simulink library "AeroLib"  (Simulink 6.0)
settings: Solver=ode45  SolverMode=SingleTasking  StartTime=0.0  StopTime=10.0  RelTol=1e-3
undefined symbols (not defined in the file): Aero, Ap, Atm, Control, Controls, Eng, Flight_cg, Flight_DamperON, Flight_delta_isa, Flight_DeltaSpiral, Flight_InertiaSelect, Flight_ixx, Flight_ixz, Flight_iyy, Flight_izz, Flight_latitude, Flight_LoiterLenght, Flight_LoiterMode, Flight_LoiterRadius, Flight_longitude, Flight_MaxTargetPoints, Flight_SensorsON, Flight_TimeStep, Flight_TowerWind_X, Flight_TowerWind_Y, Flight_TowerWind_Z, Flight_TowerWindON, Flight_Trimming, Flight_TurbON, Flight_weight, Flight_WindGustON, Flight_WindShearON, Flight_ycg, Flight_zcg, Geom, Lgear, Mass, PEG_CDwbnp, PEG_CLht, PEG_CLht_elev, PEG_CLwbnp, PEG_CMht, PEG_CMwbnp, PEG_CNbeta, PEG_CNr, PEG_CNrud, PEG_CRail, PEG_CRbeta, PEG_CRp, PEG_CRrud, PEG_CYbeta, PEG_CYrud, pow, Sensors
libraries: AeroLib x133, simulink3 x49, simulink x37, aerospace x11
(part 3 of 7)

== system AeroLib/Propulsion/Piston_Engine ==
  FeedBack : Inport  Port=1  LatchInput=off
  From_Atmos : Inport  Port=2  LatchInput=off
  Throttle : Inport  Port=3  LatchInput=off
  From_Reset : Inport  Port=4  LatchInput=off
  Fuel_Cut : Inport  Port=5  LatchInput=off
  AVGAS100_Density : Gain  Gain=0.7  SaturateOnIntegerOverflow=on
  Altitude_delta : Fcn  Expr=1.11*sqrt(1/u(1))*u(2) - 0.11
  Bus Selector2 : BusSelector  DialogController=Simulink.DDGSource_Bus  OutputSignals=T_T0,P_P0
  Constant3 : Constant  Value=0
  Constant5 : Constant  Value=0
  Constant6 : Constant  Value=Eng.Fuel.mass
  Fcn : Fcn  Expr=1-u
  Fuel_Flow_Kgps : simulink/Lookup Tables/Interpolation (n-D) using PreLookup  numDimsPopupSelect=1  explicitNumDims=2  table=Eng.Cons  interpMethod=Linear  extrapMethod=Linear  rangeErrorMode=None  NumSelectionDims=0
  Max_Available_Power : simulink/Lookup Tables/Interpolation (n-D) using PreLookup  numDimsPopupSelect=1  explicitNumDims=2  table=Eng.power  interpMethod=Linear  extrapMethod=Linear  rangeErrorMode=None  NumSelectionDims=0
  Mux5 : Mux  Inputs=2
  Product1 : Product  SaturateOnIntegerOverflow=on  InputSameDT=on
  Product2 : Product  SaturateOnIntegerOverflow=on  InputSameDT=on
  Rot_par_min : Fcn  Expr=Eng.MaxRpm*u
  Saturation : Saturate  UpperLimit=Eng.MaxRpm  LowerLimit=Eng.MinRpm
  Stateless_LimIntegrator : AeroLib/AMS_StatelessFilters/Stateless_LimIntegrator
  Sum : Sum  Inputs=++|  SaturateOnIntegerOverflow=on  InputSameDT=on
  Turn : simulink/Lookup Tables/PreLookup Index Search  bpData=Eng.Rpm  searchMode=Binary Search  cacheBpFlag=off  outputFlag=off  IndexDataType=uint32  extrapMode=Linear Extrapolation  rangeErrorMode=None
  Avail_Power : Outport
  RPM : Outport  Port=2
  Fuel_Mass : Outport  Port=3
  wires:
  Fcn/1 -> Product1/2
  Fuel_Flow_Kgps/1 -> Product1/1
  Product1/1 -> AVGAS100_Density/1
  Fuel_Cut/1 -> Fcn/1
  Turn/1 -> Max_Available_Power/1, Fuel_Flow_Kgps/1
  Mux5/1 -> Altitude_delta/1
  Max_Available_Power/1 -> Product2/1
  Altitude_delta/1 -> Product2/2
  Bus Selector2/2 -> Mux5/2  "<P_P0>"
  Bus Selector2/1 -> Mux5/1  "<T_T0>"
  Throttle/1 -> Rot_par_min/1
  Saturation/1 -> Turn/1, RPM/1
  Rot_par_min/1 -> Sum/2
  Sum/1 -> Saturation/1
  FeedBack/1 -> Sum/1
  Product2/1 -> Avail_Power/1
  From_Atmos/1 -> Bus Selector2/1
  AVGAS100_Density/1 -> Stateless_LimIntegrator/3
  Constant3/1 -> Stateless_LimIntegrator/2
  From_Reset/1 -> Stateless_LimIntegrator/1
  Stateless_LimIntegrator/1 -> Fuel_Mass/1
  Constant5/1 -> Stateless_LimIntegrator/4
  Constant6/1 -> Stateless_LimIntegrator/5

== system AeroLib/Propulsion/Piston_Engine_Propeller ==
  From_Atmos : Inport  Port=1  LatchInput=off
  Throttle : Inport  Port=2  LatchInput=off
  From_Reset : Inport  Port=3  LatchInput=off
  Fuel_Cut : Inport  Port=4  LatchInput=off
  Air_Dens : Fcn  Expr=2*u(2)/u(1)^2
  Bus Selector2 : BusSelector  DialogController=Simulink.DDGSource_Bus  OutputSignals=Mach,TAS,DynPres_P
  Fcn : Fcn  Expr=1-u
  Fixed_Pitch_Propeller : AeroLib/Propulsion/Fixed_Pitch_Propeller  reduc=Eng.Prop.reduc  prop_diam=Eng.Prop.diam
  Gain1 : Gain  Gain=Atm.grav  SaturateOnIntegerOverflow=on
  Mux6 : Mux  Inputs=2
  Piston_Engine : AeroLib/Propulsion/Piston_Engine
  Power_Limit : Subsystem
  Product : Product  SaturateOnIntegerOverflow=on  InputSameDT=on
  Propeller_Power_Demand : AeroLib/Propulsion/Propeller_Power_Demand  D=Eng.Prop.diam
  Thrust_N : Outport
  RPM : Outport  Port=2
  Efficiency_coef : Outport  Port=3
  Fuel_Mass : Outport  Port=4
  wires:
  Gain1/1 -> Thrust_N/1
  Fcn/1 -> Product/2
  Product/1 -> Gain1/1
  Fuel_Cut/1 -> Piston_Engine/5, Fcn/1
  From_Reset/1 -> Piston_Engine/4
  Piston_Engine/3 -> Fuel_Mass/1
  Bus Selector2/1 -> Fixed_Pitch_Propeller/2  "<Mach>"
  Bus Selector2/3 -> Mux6/2  "<DynPres_P>"
  Bus Selector2/2 -> Fixed_Pitch_Propeller/3, Mux6/1  "<TAS>"
  Piston_Engine/1 -> Power_Limit/1(Avail_Power)
  Piston_Engine/2 -> Fixed_Pitch_Propeller/1, Power_Limit/2(Rpm), RPM/1
  Throttle/1 -> Piston_Engine/3
  Power_Limit/1(Delta_Rpm) -> Piston_Engine/1
  Propeller_Power_Demand/1 -> Power_Limit/3(Power_Demand)
  Fixed_Pitch_Propeller/3 -> Propeller_Power_Demand/3
  Fixed_Pitch_Propeller/2 -> Propeller_Power_Demand/2
  Fixed_Pitch_Propeller/1 -> Propeller_Power_Demand/1
  Mux6/1 -> Air_Dens/1
  From_Atmos/1 -> Piston_Engine/2, Bus Selector2/1
  Propeller_Power_Demand/2 -> Product/1
  Fixed_Pitch_Propeller/4 -> Efficiency_coef/1
  Air_Dens/1 -> Propeller_Power_Demand/4

== system AeroLib/Propulsion/Piston_Engine_Propeller_system ==
  note: These blocks is included to allow model to be used
      | with DINAMO.
      | DINAMO's Trim capabilities need the model
      | to contain a twin engine type of propulsion system.
  From_Atmos : Inport  Port=1  LatchInput=off
  From_Ctrl : Inport  Port=2  LatchInput=off
  From_Inputs : Inport  Port=3  LatchInput=off
  From_Reset : Inport  Port=4  LatchInput=off
  Booster : AeroLib/Propulsion/Booster  Booster_Time=Eng.Booster.Time  Xpos=Geom.Eng.Booster.Xpos  Ypos=Geom.Eng.Booster.Ypos  Zpos=Geom.Eng.Booster.Zpos  Booster_Thrust=Eng.Booster.Thrust  pitch=Geom.Eng.Booster.pitch
  Bus Creator : BusCreator  DialogController=Simulink.DDGSource_Bus  Inputs=16
  Bus Selector2 : BusSelector  DialogController=Simulink.DDGSource_Bus  OutputSignals=DynPres_P
  Bus Selector3 : BusSelector  DialogController=Simulink.DDGSource_Bus  OutputSignals=FuelCut_LH,FuelCut_RH,BoosterON
  Engine_Transient : AeroLib/Propulsion/Engine_Transient
  Fantom_Engine : Gain  Gain=eps  SaturateOnIntegerOverflow=on
  Fantom_Engine1 : Gain  Gain=eps  SaturateOnIntegerOverflow=on
  Piston_Engine_Propeller_LH : AeroLib/Propulsion/Piston_Engine_Propeller
  Piston_Engine_Propeller_RH : AeroLib/Propulsion/Piston_Engine_Propeller
  Terminator2 : Terminator
  Terminator3 : Terminator
  Thrust_Components : AeroLib/Propulsion/Thrust_Components  grav=Atm.grav  Sw=Geom.Wing.sw  Xpos=Geom.Eng.Xpos  Ypos=Geom.Eng.Ypos  Zpos=Geom.Eng.Zpos  pitch=Geom.Eng.pitch  toeout=Geom.Eng.toeout
  Prop_Out : Outport
  wires:
  Bus Selector2/1 -> Thrust_Components/4  "<DynPres_P>"
  Thrust_Components/12 -> Bus Creator/14  "RH_Throttle"
  Thrust_Components/11 -> Bus Creator/13  "LH_Throttle"
  Piston_Engine_Propeller_LH/4 -> Thrust_Components/2
  From_Atmos/1 -> Piston_Engine_Propeller_RH/1, Piston_Engine_Propeller_LH/1, Bus Selector2/1
  Thrust_Components/9 -> Bus Creator/11  "Thrust_N"
  Thrust_Components/10 -> Bus Creator/12  "DeltaThr"
  Thrust_Components/8 -> Bus Creator/10  "Thrust_Kgf"
  Thrust_Components/7 -> Bus Creator/9  "CT"
  Thrust_Components/6 -> Bus Creator/8  "Nthrust"
  Thrust_Components/5 -> Bus Creator/7  "Mthrust"
  Bus Creator/1 -> Prop_Out/1
  Thrust_Components/1 -> Bus Creator/3  "Xthrust"
  Thrust_Components/4 -> Bus Creator/6  "Lthrust"
  Thrust_Components/3 -> Bus Creator/5  "Zthrust"
  Thrust_Components/2 -> Bus Creator/4  "Ythrust"
  From_Ctrl/1 -> Engine_Transient/1
  From_Inputs/1 -> Bus Selector3/1
  From_Reset/1 -> Piston_Engine_Propeller_LH/3, Piston_Engine_Propeller_RH/3, Booster/2, Engine_Transient/2
  Piston_Engine_Propeller_RH/1 -> Fantom_Engine/1
  Piston_Engine_Propeller_RH/4 -> Fantom_Engine1/1
  Piston_Engine_Propeller_RH/3 -> Terminator2/1
  Booster/1 -> Thrust_Components/8
  Booster/2 -> Bus Creator/16  "StopBooster"
  Engine_Transient/1 -> Piston_Engine_Propeller_LH/2, Thrust_Components/3
  Engine_Transient/2 -> Piston_Engine_Propeller_RH/2, Thrust_Components/7
  Piston_Engine_Propeller_LH/1 -> Thrust_Components/1
  Fantom_Engine/1 -> Thrust_Components/5
  Thrust_Components/13 -> Bus Creator/15  "Fuel_Mass"
  Fantom_Engine1/1 -> Thrust_Components/6
  Piston_Engine_Propeller_LH/2 -> Bus Creator/1  "Rpm_Eng"
  Piston_Engine_Propeller_LH/3 -> Bus Creator/2  "Effic_Prop"
  Bus Selector3/1 -> Piston_Engine_Propeller_LH/4  "<FuelCut_LH>"
  Bus Selector3/2 -> Piston_Engine_Propeller_RH/4  "<FuelCut_RH>"
  Bus Selector3/3 -> Booster/1  "<BoosterON>"
  Piston_Engine_Propeller_RH/2 -> Terminator3/1

== system AeroLib/Propulsion/Propeller_Power_Demand ==
  note: in kg/m3
  note: in hp
  Thrust_coef : Inport  Port=1  LatchInput=off
  Power_coef : Inport  Port=2  LatchInput=off
  Propeller_rps : Inport  Port=3  LatchInput=off
  Air_density : Inport  Port=4  LatchInput=off
  Mux2 : Mux
  N-->Kg : Gain  Gain=1/Atm.grav  SaturateOnIntegerOverflow=on
  Propeller_Power_Demand : Fcn  Expr=u(2)*u(4)*u(3)^3*D^5/75
  Propeller_Trust : Fcn  Expr=u(1)*u(4)*u(3)^2*D^4
  Power_demand : Outport
  Thrust_kgf : Outport  Port=2
  wires:
  Mux2/1 -> Propeller_Trust/1, Propeller_Power_Demand/1
  Thrust_coef/1 -> Mux2/1
  Power_coef/1 -> Mux2/2
  Propeller_rps/1 -> Mux2/3
  Air_density/1 -> N-->Kg/1
  Propeller_Power_Demand/1 -> Power_demand/1
  Propeller_Trust/1 -> Thrust_kgf/1
  N-->Kg/1 -> Mux2/4

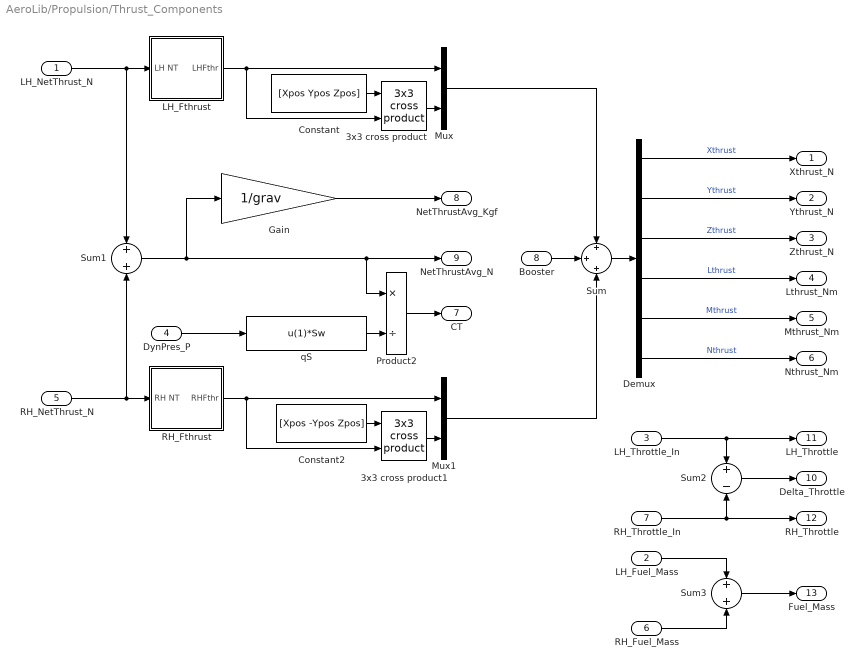
== system AeroLib/Propulsion/Thrust_Components ==
  LH_NetThrust_N : Inport  Port=1  LatchInput=off
  LH_Fuel_Mass : Inport  Port=2  LatchInput=off
  LH_Throttle_In : Inport  Port=3  LatchInput=off
  DynPres_P : Inport  Port=4  LatchInput=off
  RH_NetThrust_N : Inport  Port=5  LatchInput=off
  RH_Fuel_Mass : Inport  Port=6  LatchInput=off
  RH_Throttle_In : Inport  Port=7  LatchInput=off
  Booster : Inport  Port=8  LatchInput=off
  3x3 cross product : aerospace/Axes Transformations/3x3 cross product
  3x3 cross product1 : aerospace/Axes Transformations/3x3 cross product
  Constant : Constant  Value=[Xpos Ypos Zpos]
  Constant2 : Constant  Value=[Xpos -Ypos Zpos]
  Demux : Demux  Outputs=6
  Gain : Gain  Gain=1/grav  SaturateOnIntegerOverflow=on
  LH_Fthrust : Subsystem
  Mux : Mux  Inputs=2
  Mux1 : Mux  Inputs=2
  Product2 : Product  Inputs=*/  SaturateOnIntegerOverflow=on  InputSameDT=on
  RH_Fthrust : Subsystem
  Sum : Sum  Inputs=+|+|+  SaturateOnIntegerOverflow=on  InputSameDT=on
  Sum1 : Sum  SaturateOnIntegerOverflow=on  InputSameDT=on
  Sum2 : Sum  Inputs=+-  SaturateOnIntegerOverflow=on  InputSameDT=on
  Sum3 : Sum  SaturateOnIntegerOverflow=on  InputSameDT=on
  qS : Fcn  Expr=u(1)*Sw
  Xthrust_N : Outport
  Ythrust_N : Outport  Port=2
  Zthrust_N : Outport  Port=3
  Lthrust_Nm : Outport  Port=4
  Mthrust_Nm : Outport  Port=5
  Nthrust_Nm : Outport  Port=6
  CT : Outport  Port=7
  NetThrustAvg_Kgf : Outport  Port=8
  NetThrustAvg_N : Outport  Port=9
  Delta_Throttle : Outport  Port=10
  LH_Throttle : Outport  Port=11
  RH_Throttle : Outport  Port=12
  Fuel_Mass : Outport  Port=13
  wires:
  Sum3/1 -> Fuel_Mass/1
  RH_Fuel_Mass/1 -> Sum3/2
  LH_Fuel_Mass/1 -> Sum3/1
  Gain/1 -> NetThrustAvg_Kgf/1
  DynPres_P/1 -> qS/1
  RH_Throttle_In/1 -> RH_Throttle/1, Sum2/2
  LH_Throttle_In/1 -> LH_Throttle/1, Sum2/1
  Sum1/1 -> Gain/1, Product2/1, NetThrustAvg_N/1
  Booster/1 -> Sum/2
  Constant2/1 -> 3x3 cross product1/1
  3x3 cross product1/1 -> Mux1/2
  Mux1/1 -> Sum/3
  RH_NetThrust_N/1 -> Sum1/2, RH_Fthrust/1(RH NT)
  RH_Fthrust/1(RHFthr) -> 3x3 cross product1/2, Mux1/1
  Sum2/1 -> Delta_Throttle/1
  Demux/1 -> Xthrust_N/1  "Xthrust"
  Demux/6 -> Nthrust_Nm/1  "Nthrust"
  Demux/5 -> Mthrust_Nm/1  "Mthrust"
  Demux/4 -> Lthrust_Nm/1  "Lthrust"
  Demux/3 -> Zthrust_N/1  "Zthrust"
  Demux/2 -> Ythrust_N/1  "Ythrust"
  Constant/1 -> 3x3 cross product/1
  3x3 cross product/1 -> Mux/2
  Mux/1 -> Sum/1
  Product2/1 -> CT/1
  qS/1 -> Product2/2
  LH_NetThrust_N/1 -> Sum1/1, LH_Fthrust/1(LH NT)
  LH_Fthrust/1(LHFthr) -> Mux/1, 3x3 cross product/2
  Sum/1 -> Demux/1

== system AeroLib/Propulsion/Twin_Jet_Engine_system ==
  From_Atmos : Inport  Port=1  LatchInput=off
  From_Ctrl : Inport  Port=2  LatchInput=off
  From_Inputs : Inport  Port=3  LatchInput=off
  From_Reset : Inport  Port=4  LatchInput=off
  Booster : AeroLib/Propulsion/Booster  Booster_Time=Eng.Booster.Time  Xpos=Geom.Eng.Booster.Xpos  Ypos=Geom.Eng.Booster.Ypos  Zpos=Geom.Eng.Booster.Zpos  Booster_Thrust=Eng.Booster.Thrust  pitch=Geom.Eng.Booster.pitch
  Bus Selector1 : BusSelector  DialogController=Simulink.DDGSource_Bus  OutputSignals=DynPres_P
  Bus Selector3 : BusSelector  DialogController=Simulink.DDGSource_Bus  OutputSignals=FuelCut_LH,FuelCut_RH,BoosterON
  Engine_Transient : AeroLib/Propulsion/Engine_Transient
  Jet_Engine_LH : AeroLib/Propulsion/Jet_Engine
  Jet_Engine_RH : AeroLib/Propulsion/Jet_Engine
  Mux : Mux  Inputs=14
  Thrust_Components : AeroLib/Propulsion/Thrust_Components  grav=Atm.grav  Sw=Geom.Wing.sw  Xpos=Geom.Eng.Xpos  Ypos=Geom.Eng.Ypos  Zpos=Geom.Eng.Zpos  pitch=Geom.Eng.pitch  toeout=Geom.Eng.toeout
  Prop_Out : Outport
  wires:
  From_Atmos/1 -> Jet_Engine_LH/2, Jet_Engine_RH/2, Bus Selector1/1
  Engine_Transient/2 -> Jet_Engine_RH/1
  From_Inputs/1 -> Bus Selector3/1
  Booster/2 -> Mux/14  "StopBooster"
  Thrust_Components/2 -> Mux/2  "Ythrust"
  Thrust_Components/3 -> Mux/3  "Zthrust"
  Thrust_Components/4 -> Mux/4  "Lthrust"
  Thrust_Components/1 -> Mux/1  "Xthrust"
  Thrust_Components/5 -> Mux/5  "Mthrust"
  Thrust_Components/6 -> Mux/6  "Nthrust"
  Thrust_Components/7 -> Mux/7  "CT"
  Thrust_Components/8 -> Mux/8  "Thrust_Kgf"
  Thrust_Components/10 -> Mux/10  "DeltaThr"
  Thrust_Components/9 -> Mux/9  "Thrust_N"
  Mux/1 -> Prop_Out/1
  Jet_Engine_RH/3 -> Thrust_Components/7
  Jet_Engine_RH/1 -> Thrust_Components/5
  Booster/1 -> Thrust_Components/8
  Jet_Engine_LH/3 -> Thrust_Components/3
  Jet_Engine_LH/1 -> Thrust_Components/1
  Thrust_Components/13 -> Mux/13  "Fuel_Mass"
  Jet_Engine_LH/2 -> Thrust_Components/2
  Jet_Engine_RH/2 -> Thrust_Components/6
  From_Ctrl/1 -> Engine_Transient/1
  From_Reset/1 -> Jet_Engine_RH/4, Jet_Engine_LH/4, Booster/2, Engine_Transient/2
  Engine_Transient/1 -> Jet_Engine_LH/1
  Thrust_Components/11 -> Mux/11  "RH_Throttle"
  Bus Selector3/1 -> Jet_Engine_LH/3  "<FuelCut_LH>"
  Bus Selector3/2 -> Jet_Engine_RH/3  "<FuelCut_RH>"
  Bus Selector3/3 -> Booster/1  "<BoosterON>"
  Thrust_Components/12 -> Mux/12  "LH_Throttle"
  Bus Selector1/1 -> Thrust_Components/4  "<DynPres_P>"

== system AeroLib/Propulsion/Variable_Pitch_Propeller ==
  note: deg
  RPM : Inport  Port=1  LatchInput=off
  Mach : Inport  Port=2  LatchInput=off
  TAS_mps : Inport  Port=3  LatchInput=off
  PropPitch : Inport  Port=4  LatchInput=off
  Advance_Ratio : Fcn  Expr=u(1)/(prop_diam*u(2))
  Beta : simulink/Lookup Tables/PreLookup Index Search  bpData=Eng.Prop.Beta  searchMode=Binary Search  cacheBpFlag=off  outputFlag=off  IndexDataType=uint32  extrapMode=Linear Extrapolation  rangeErrorMode=None
  CP : simulink/Lookup Tables/Interpolation (n-D) using PreLookup  numDimsPopupSelect=2  explicitNumDims=2  table=Eng.Prop.Cp  interpMethod=Linear  extrapMethod=Linear  rangeErrorMode=None  NumSelectionDims=0
  CT : simulink/Lookup Tables/Interpolation (n-D) using PreLookup  numDimsPopupSelect=2  explicitNumDims=2  table=Eng.Prop.Ct  interpMethod=Linear  extrapMethod=Linear  rangeErrorMode=None  NumSelectionDims=0
  J : simulink/Lookup Tables/PreLookup Index Search  bpData=Eng.Prop.J  searchMode=Binary Search  cacheBpFlag=off  outputFlag=off  IndexDataType=uint32  extrapMode=Linear Extrapolation  rangeErrorMode=None
  Mach_Number_Effect : Subsystem
  Mux1 : Mux  Inputs=2
  Product1 : Product  Inputs=**/  SaturateOnIntegerOverflow=on  InputSameDT=on
  Product2 : Product  Inputs=*/  SaturateOnIntegerOverflow=on  InputSameDT=on
  Product4 : Product  SaturateOnIntegerOverflow=on  InputSameDT=on
  Reduction : Gain  Gain=1/reduc/60  SaturateOnIntegerOverflow=on
  Thrust_coef : Outport
  Power_coef : Outport  Port=2
  Propeller_rps : Outport  Port=3
  Efficiency_coef : Outport  Port=4
  wires:
  PropPitch/1 -> Mach_Number_Effect/5(Prop_Pitch_deg), Beta/1
  Beta/1 -> ?
  J/1 -> CT/1, CP/1
  Mux1/1 -> Advance_Ratio/1
  CP/1 -> Product2/1
  Reduction/1 -> Mux1/2, Propeller_rps/1, Mach_Number_Effect/2(Prop_rps)
  TAS_mps/1 -> Mux1/1, Mach_Number_Effect/3(TAS)
  RPM/1 -> Reduction/1
  Product1/1 -> Efficiency_coef/1
  Mach/1 -> Mach_Number_Effect/4(Mach)
  Product2/1 -> Power_coef/1, Product1/3
  Mach_Number_Effect/2(Kcp) -> Product2/2
  CT/1 -> Product4/1
  Product4/1 -> Product1/1, Thrust_coef/1
  Mach_Number_Effect/1(Km) -> Product4/2
  Advance_Ratio/1 -> Product1/2, J/1, Mach_Number_Effect/1(J)

== system AeroLib/Sensors/Air_Data_Computer ==
  From_Atmos : Inport  Port=1  LatchInput=off
  From_Reset : Inport  Port=2  LatchInput=off
  Bus Selector1 : BusSelector  DialogController=Simulink.DDGSource_Bus  OutputSignals=Pamb_P,DynPres_P,OAT_degC,PresAlt_ft
  Gain2 : Gain  SaturateOnIntegerOverflow=on
  Gain3 : Gain  SaturateOnIntegerOverflow=on
  Gain4 : Gain  SaturateOnIntegerOverflow=on
  Mux : Mux
  Mux1 : Mux  Inputs=3
  SensorsOFF : Subsystem
  Simple_Sensor : AeroLib/Sensors/Simple_Sensor  Var=Sensors.ADC.Var  Seed=Sensors.ADC.Seed  Max=60000  Min=-300  Time_Const=Sensors.ADC.TimeConst
  Sum : Sum  Inputs=++|  SaturateOnIntegerOverflow=on  InputSameDT=on
  Switch : Switch  Threshold=0.5  SaturateOnIntegerOverflow=on  InputSameDT=on
  Ts*Ps/Pt : Fcn  Expr=u(3) * u(2) / u(1)
  ADC_Out : Outport
  wires:
  Simple_Sensor/1 -> Switch/3
  From_Reset/1 -> Simple_Sensor/3
  Switch/1 -> Mux/4  "ADC_PresAlt_ft"
  SensorsOFF/1(SensorsOFF) -> Switch/2
  Bus Selector1/1 -> Sum/1, Gain2/1, Mux1/2  "<Pamb_P>"
  Ts*Ps/Pt/1 -> Gain3/1
  Mux1/1 -> Ts*Ps/Pt/1
  Bus Selector1/3 -> Mux1/3  "<OAT_degC>"
  Bus Selector1/2 -> Sum/2  "<DynPres_P>"
  Sum/1 -> Mux1/1, Gain4/1  "Pt"
  Gain2/1 -> Mux/1  "ADC_Pamb_P"
  Gain3/1 -> Mux/3  "ADC_OAT_degC"
  Gain4/1 -> Mux/2  "ADC_DynlPres_P"
  Mux/1 -> ADC_Out/1
  From_Atmos/1 -> Bus Selector1/1
  Bus Selector1/4 -> Switch/1, Simple_Sensor/1, Simple_Sensor/2  "<PresAlt_ft>"

== system AeroLib/Sensors/Flight_System_Computer ==
  From_IRU : Inport  Port=1  LatchInput=off
  From_GPS : Inport  Port=2  LatchInput=off
  From_ADC : Inport  Port=3  LatchInput=off
  Bus Creator : BusCreator  DialogController=Simulink.DDGSource_Bus  Inputs=26
  Bus Selector1 : BusSelector  DialogController=Simulink.DDGSource_Bus  OutputSignals=IRU_Alpha,IRU_Beta,IRU_KIAS,IRU_TAS_kt,IRU_RadarAlt_ft,IRU_Phi_deg,IRU_Q_degps,IRU_P_degps,IRU_R_degps,IRU_LongAcc_g,IRU_NormAcc_g,IRU_LatAcc_g,IRU_Theta_deg,IRU_HeadMag_deg,IRU_FPath_deg
  Bus Selector4 : BusSelector  DialogController=Simulink.DDGSource_Bus  OutputSignals=IRU_Xdist_m,IRU_Ydist_m,IRU_Latitude_deg,IRU_Longitude_deg,IRU_GeodHeight_m,IRU_VN_kt,IRU_VE_kt,IRU_VD_mps,IRU_GrSpeed_kt,IRU_TrackMag_deg
  Bus Selector5 : BusSelector  DialogController=Simulink.DDGSource_Bus  OutputSignals=GPS_Xdist_m,GPS_Ydist_m,GPS_Latitude_deg,GPS_Longitude_deg,GPS_GeodHeight_m,GPS_VN_kt,GPS_VE_kt,GPS_VD_mps,GPS_Vground_kt,GPS_Track_deg
  Bus Selector6 : BusSelector  DialogController=Simulink.DDGSource_Bus  OutputSignals=ADC_PresAlt_ft
  Bus Selector7 : BusSelector  DialogController=Simulink.DDGSource_Bus  OutputSignals=IRU_PresAlt_ft
  Demux : Demux  Outputs=10
  Gain : Gain  Gain=Kins  SaturateOnIntegerOverflow=on
  Gain1 : Gain  Gain=0.5  SaturateOnIntegerOverflow=on
  Gain2 : Gain  Gain=Kgps  SaturateOnIntegerOverflow=on
  Mux1 : Mux  Inputs=10
  Mux2 : Mux  Inputs=10
  Sum : Sum  Inputs=|++  SaturateOnIntegerOverflow=on  InputSameDT=on
  Sum1 : Sum  Inputs=|++  SaturateOnIntegerOverflow=on  InputSameDT=on
  FSC_Out : Outport
  wires:
  Bus Selector1/15 -> Bus Creator/26  "<IRU_FPath_deg>"
  Bus Selector1/14 -> Bus Creator/25  "<IRU_HeadMag_deg>"
  Bus Selector1/13 -> Bus Creator/24  "<IRU_Theta_deg>"
  Bus Creator/1 -> FSC_Out/1
  Bus Selector1/12 -> Bus Creator/23  "<IRU_LatAcc_g>"
  Bus Selector1/11 -> Bus Creator/22  "<IRU_NormAcc_g>"
  Bus Selector1/10 -> Bus Creator/21  "<IRU_LongAcc_g>"
  Bus Selector1/9 -> Bus Creator/20  "<IRU_R_degps>"
  Bus Selector1/8 -> Bus Creator/19  "<IRU_P_degps>"
  Bus Selector1/7 -> Bus Creator/18  "<IRU_Q_degps>"
  Bus Selector1/6 -> Bus Creator/17  "<IRU_Phi_deg>"
  Bus Selector1/5 -> Bus Creator/16  "<IRU_RadarAlt_ft>"
  Bus Selector1/4 -> Bus Creator/15  "<IRU_TAS_kt>"
  Bus Selector1/3 -> Bus Creator/14  "<IRU_KIAS>"
  Bus Selector1/2 -> Bus Creator/13  "<IRU_Beta>"
  Bus Selector1/1 -> Bus Creator/12  "<IRU_Alpha>"
  Gain1/1 -> Bus Creator/1  "FSC_Altitude_ft"
  Demux/10 -> Bus Creator/11  "FSC_TrackMag_deg"
  Demux/9 -> Bus Creator/10  "FSC_GrSpeed_kt"
  Demux/8 -> Bus Creator/9  "FSC_VD_mps"
  Demux/7 -> Bus Creator/8  "FSC_VE_kt"
  Demux/6 -> Bus Creator/7  "FSC_VN_kt"
  Demux/5 -> Bus Creator/6  "FSC_GeodHeight_m"
  Demux/4 -> Bus Creator/5  "FSC_Longitude_deg"
  Demux/3 -> Bus Creator/4  "FSC_Latitude_deg"
  Demux/2 -> Bus Creator/3  "FSC_Ydist_m"
  Demux/1 -> Bus Creator/2  "FSC_Xdist_m"
  Sum/1 -> Demux/1
  Sum1/1 -> Gain1/1
  Bus Selector7/1 -> Sum1/2  "<IRU_PresAlt_ft>"
  Bus Selector6/1 -> Sum1/1  "<ADC_PresAlt_ft>"
  Bus Selector4/10 -> Mux2/10  "<IRU_TrackMag_deg>"
  Bus Selector4/9 -> Mux2/9  "<IRU_GrSpeed_kt>"
  Bus Selector4/8 -> Mux2/8  "<IRU_VD_mps>"
  Bus Selector4/7 -> Mux2/7  "<IRU_VE_kt>"
  Bus Selector4/6 -> Mux2/6  "<IRU_VN_kt>"
  Bus Selector4/5 -> Mux2/5  "<IRU_GeodHeight_m>"
  Bus Selector4/4 -> Mux2/4  "<IRU_Longitude_deg>"
  Bus Selector4/3 -> Mux2/3  "<IRU_Latitude_deg>"
  Bus Selector4/2 -> Mux2/2  "<IRU_Ydist_m>"
  Bus Selector4/1 -> Mux2/1  "<IRU_Xdist_m>"
  Bus Selector5/10 -> Mux1/10  "<GPS_Track_deg>"
  Bus Selector5/9 -> Mux1/9  "<GPS_Vground_kt>"
  Bus Selector5/8 -> Mux1/8  "<GPS_VD_mps>"
  Bus Selector5/7 -> Mux1/7  "<GPS_VE_kt>"
  Bus Selector5/6 -> Mux1/6  "<GPS_VN_kt>"
  Bus Selector5/5 -> Mux1/5  "<GPS_GeodHeight_m>"
  Bus Selector5/4 -> Mux1/4  "<GPS_Longitude_deg>"
  Bus Selector5/3 -> Mux1/3  "<GPS_Latitude_deg>"
  Bus Selector5/2 -> Mux1/2  "<GPS_Ydist_m>"
  Bus Selector5/1 -> Mux1/1  "<GPS_Xdist_m>"
  Gain2/1 -> Sum/2
  Gain/1 -> Sum/1
  Mux1/1 -> Gain2/1
  Mux2/1 -> Gain/1
  From_IRU/1 -> Bus Selector1/1, Bus Selector7/1, Bus Selector4/1
  From_ADC/1 -> Bus Selector6/1
  From_GPS/1 -> Bus Selector5/1

== system AeroLib/Sensors/Gauss_Markov ==
  Reset : Inport  Port=1  LatchInput=off
  Constant : Constant  Value=0
  Gain : Gain  Orientation=left  Gain=1/tau  SaturateOnIntegerOverflow=on
  Stateless_Integrator : AeroLib/AMS_StatelessFilters/Stateless_Integrator
  Sum : Sum  Inputs=|+-  SaturateOnIntegerOverflow=on  InputSameDT=on
  White Noise : RandomNumber  Variance=Var  Seed=Seed  SampleTime=Flight_TimeStep
  Noise : Outport
  wires:
  Reset/1 -> Stateless_Integrator/1
  Constant/1 -> Stateless_Integrator/2
  White Noise/1 -> Sum/1
  Sum/1 -> Stateless_Integrator/3
  Stateless_Integrator/1 -> Noise/1, Gain/1
  Gain/1 -> Sum/2

== system AeroLib/Sensors/Global_Positioning_System ==
  Latitude : Inport  Port=1  LatchInput=off
  Longitude : Inport  Port=2  LatchInput=off
  GeodHeight : Inport  Port=3  LatchInput=off
  VN_kt : Inport  Port=4  LatchInput=off
  VE_kt : Inport  Port=5  LatchInput=off
  VD_mps : Inport  Port=6  LatchInput=off
  Xdist_m : Inport  Port=7  LatchInput=off
  Ydist_m : Inport  Port=8  LatchInput=off
  Track_deg : Inport  Port=9  LatchInput=off
  From_Reset : Inport  Port=10  LatchInput=off
  Bus Creator : BusCreator  DialogController=Simulink.DDGSource_Bus  Inputs=10
  Clock : Clock
      settings: Decimation=10
  Constant : Constant  Value=Flight_Trimming
  Demux : Demux  Outputs=9
  Fcn : Fcn  Expr=u <= max(Time_delay)
  Fcn1 : Fcn  Expr=sqrt(u(4)^2 + u(5)^2)
  Mux : Mux  Inputs=9
  SensorsOFF : Subsystem
  Simple_GPS : Subsystem
  Switch : Switch  Threshold=0.5  SaturateOnIntegerOverflow=on  InputSameDT=on
  Switch1 : Switch  Threshold=0.5  SaturateOnIntegerOverflow=on  InputSameDT=on
  or : Logic  Operator=OR
  GPS_Out : Outport
  wires:
  From_Reset/1 -> Simple_GPS/2("From_Reset ")
  Switch1/1 -> Fcn1/1, Demux/1
  Switch/1 -> Switch1/3
  SensorsOFF/1(SensorsOFF) -> Switch1/2
  Clock/1 -> Fcn/1
  Constant/1 -> or/1  "DT"
  Fcn/1 -> or/2
  or/1 -> Switch/2
  Latitude/1 -> Mux/1
  Longitude/1 -> Mux/2
  GeodHeight/1 -> Mux/3
  VN_kt/1 -> Mux/4
  VE_kt/1 -> Mux/5
  VD_mps/1 -> Mux/6
  Simple_GPS/1(GPS_Out) -> Switch/3
  Demux/6 -> Bus Creator/6  "GPS_VD_mps"
  Demux/5 -> Bus Creator/5  "GPS_VE_kt"
  Demux/4 -> Bus Creator/4  "GPS_VN_kt"
  Demux/3 -> Bus Creator/3  "GPS_GeodHeight_m"
  Demux/2 -> Bus Creator/2  "GPS_Longitude_deg"
  Demux/1 -> Bus Creator/1  "GPS_Latitude_deg"
  Mux/1 -> Simple_GPS/1(Measured_In), Switch1/1, Switch/1
  Bus Creator/1 -> GPS_Out/1
  Fcn1/1 -> Bus Creator/10  "GPS_Vground_kt"
  Xdist_m/1 -> Mux/7
  Ydist_m/1 -> Mux/8
  Demux/7 -> Bus Creator/7  "GPS_Xdist_m"
  Demux/8 -> Bus Creator/8  "GPS_Ydist_m"
  Track_deg/1 -> Mux/9
  Demux/9 -> Bus Creator/9  "GPS_Track_deg"

== system AeroLib/Sensors/Inertial_Reference_Unit ==
  From_EQM : Inport  Port=1  LatchInput=off
  From_Atmos : Inport  Port=2  LatchInput=off
  From_Reset : Inport  Port=3  LatchInput=off
  Accelerometers : Subsystem
  Airspeed_Detectors : Subsystem
  Altitude_Sensors : Subsystem
  Flow_Incidence_Angle_Sensors : Subsystem
  Gyrospopes : Subsystem
  Mux : Mux  Inputs=37
  IRU_Out : Outport
  wires:
  From_Reset/1 -> Accelerometers/2(From_Reset), Flow_Incidence_Angle_Sensors/2(From_Reset), Altitude_Sensors/3(From_Reset), Airspeed_Detectors/3(From_Reset)
  From_Atmos/1 -> Altitude_Sensors/1(From_Atmos), Airspeed_Detectors/2(From_Atmos), Flow_Incidence_Angle_Sensors/1(From_Atmos)
  Altitude_Sensors/2(IRU_RadarAlt_ft) -> Mux/37  "IRU_RadarAlt_ft"
  Altitude_Sensors/1(IRU_PresAlt_ft) -> Mux/36  "IRU_PresAlt_ft"
  Flow_Incidence_Angle_Sensors/2(IRU_Beta) -> Mux/35  "IRU_Beta"
  Flow_Incidence_Angle_Sensors/1(IRU_Alpha) -> Mux/34  "IRU_Alpha"
  Airspeed_Detectors/3(IRU_TAS_kt) -> Mux/33  "IRU_TAS_kt"
  Airspeed_Detectors/2(IRU_KIAS) -> Mux/32  "IRU_KIAS"
  Airspeed_Detectors/1(IRU_GrSpeed_kt) -> Mux/31  "IRU_GrSpeed_kt"
  Accelerometers/18(IRU_GeodHeight_m) -> Mux/30  "IRU_GeodHeight_m"
  Accelerometers/17(IRU_Longitude_deg) -> Mux/29  "IRU_Longitude_deg"
  Accelerometers/16(IRU_Latitude_deg) -> Mux/28  "IRU_Latitude_deg"
  Accelerometers/14(IRU_Xdist) -> Mux/26  "IRU_Xdist_m"
  Accelerometers/15(IRU_Ydist) -> Mux/27  "IRU_Ydist_m"
  Accelerometers/13(IRU_VD_mps) -> Mux/25  "IRU_VD_mps"
  Accelerometers/11(IRU_VN_kt) -> Mux/23  "IRU_VN_kt"
  Accelerometers/12(IRU_VE_kt) -> Mux/24  "IRU_VE_kt"
  Accelerometers/9(IRU_AlongHeadAcc_g) -> Mux/21  "IRU_AlongHeadAcc_g"
  Accelerometers/10(IRU_CrossHeadAcc_g) -> Mux/22  "IRU_CrossHeadAcc_g"
  Accelerometers/8(IRU_AbNormAcc_g) -> Mux/20  "IRU_AbNormAcc_g"
  Accelerometers/7(IRU_AlongPathAcc_g) -> Mux/19  "IRU_AlongtPath_g"
  Accelerometers/6(IRU_VertAcc_g) -> Mux/18  "IRU_VertAcc_g"
  Accelerometers/4(IRU_AlongTrackAcc_g) -> Mux/16  "IRU_AlongTrackAcc_g"
  Accelerometers/5(IRU_CrossTrackAcc_g) -> Mux/17  "IRU_CrossTrackAcc_g"
  Accelerometers/1(IRU_LongAcc_g) -> Mux/13  "IRU_LongAcc_g"
  Accelerometers/2(IRU_LatAcc_g) -> Mux/14  "IRU_LatAcc_g"
  Accelerometers/3(IRU_NormAcc_g) -> Mux/15  "IRU_NormAcc_g"
  Gyrospopes/5(IRU_R_degps) -> Mux/5  "IRU_R_degps"
  Gyrospopes/4(IRU_P_degps) -> Mux/4  "IRU_P_degps"
  Gyrospopes/3(IRU_Q_degps) -> Mux/3  "IRU_Q_degps"
  Gyrospopes/2(IRU_Phi_deg) -> Mux/2  "IRU_Phi_deg"
  Gyrospopes/1(IRU_Theta_deg) -> Mux/1  "IRU_Theta_deg"
  From_EQM/1 -> Accelerometers/1(From_EQM), Airspeed_Detectors/1(From_EQM), Altitude_Sensors/2(From_EQM), Gyrospopes/1(From_EQM)
  Gyrospopes/6(IRU_Track_deg) -> Mux/6  "IRU_Track_deg"
  Gyrospopes/7(IRU_Head_deg) -> Mux/7  "IRU_Head_deg"
  Gyrospopes/12(IRU_FPath_deg) -> Mux/12  "IRU_FPath_deg"
  Mux/1 -> IRU_Out/1
  Gyrospopes/8(IRU_TrackMag_deg) -> Mux/8  "IRU_TrackMag_deg"
  Gyrospopes/9(IRU_HeadMag_deg) -> Mux/9  "IRU_HeadMag_deg"
  Gyrospopes/10(IRU_DriftAngle_deg) -> Mux/10  "IRU_DriftAngle_deg"
  Gyrospopes/11(IRU_PlatformHead_deg) -> Mux/11  "IRU_PlatformHead_deg"

== system AeroLib/Sensors/Navigation_Sensors ==
  From_EQM : Inport  Port=1  LatchInput=off
  From_Atmos : Inport  Port=2  LatchInput=off
  From_Reset : Inport  Port=3  LatchInput=off
  Air_Data_Computer : AeroLib/Sensors/Air_Data_Computer
  Bus Selector : BusSelector  DialogController=Simulink.DDGSource_Bus  OutputSignals=Latitude,Longitude,GeodHeight,VN_kt,VE_kt,VD_mps,Xdist_m,Ydist_m,Track_deg
  Flight_System_Computer : AeroLib/Sensors/Flight_System_Computer  Kgps=Sensors.FSC.Kgps  Kins=Sensors.FSC.Kins
  Global_Positioning_System : AeroLib/Sensors/Global_Positioning_System  Time_delay=Sensors.GPS.TimeDelay  Var=Sensors.GPS.Var  Seed=Sensors.GPS.Seed  Time=Sensors.GPS.CorTime
  Inertial_Reference_Unit : AeroLib/Sensors/Inertial_Reference_Unit  PlatformDev=Sensors.IRU.PlatDev  MagDev=Sensors.IRU.MagDev
  IRU_Out : Outport
  GPS_Out : Outport  Port=2
  FSC_Out : Outport  Port=3
  wires:
  Air_Data_Computer/1 -> Flight_System_Computer/3
  Global_Positioning_System/1 -> Flight_System_Computer/2, GPS_Out/1
  Flight_System_Computer/1 -> FSC_Out/1
  Bus Selector/7 -> Global_Positioning_System/7  "<Xdist_m>"
  Bus Selector/8 -> Global_Positioning_System/8  "<Ydist_m>"
  From_Reset/1 -> Global_Positioning_System/10, Inertial_Reference_Unit/3, Air_Data_Computer/2
  Bus Selector/3 -> Global_Positioning_System/3  "<GeodHeight>"
  Bus Selector/4 -> Global_Positioning_System/4  "<VN_kt>"
  Bus Selector/5 -> Global_Positioning_System/5  "<VE_kt>"
  Bus Selector/6 -> Global_Positioning_System/6  "<VD_mps>"
  Bus Selector/2 -> Global_Positioning_System/2  "<Longitude>"
  Bus Selector/1 -> Global_Positioning_System/1  "<Latitude>"
  From_EQM/1 -> Bus Selector/1, Inertial_Reference_Unit/1
  Inertial_Reference_Unit/1 -> Flight_System_Computer/1, IRU_Out/1
  From_Atmos/1 -> Air_Data_Computer/1, Inertial_Reference_Unit/2
  Bus Selector/9 -> Global_Positioning_System/9  "<Track_deg>"

== system AeroLib/Sensors/Random Walk ==
  Reset : Inport  Port=1  LatchInput=off
  Constant : Constant  Value=0
  Stateless_Integrator : AeroLib/AMS_StatelessFilters/Stateless_Integrator
  White Noise : RandomNumber  Variance=Var  Seed=Seed  SampleTime=Flight_TimeStep
  Noise : Outport
  wires:
  Reset/1 -> Stateless_Integrator/1
  Constant/1 -> Stateless_Integrator/2
  White Noise/1 -> Stateless_Integrator/3
  Stateless_Integrator/1 -> Noise/1

== system AeroLib/Sensors/Simple_Sensor ==
  Meas_In : Inport  Port=1  LatchInput=off
  X0 : Inport  Port=2  LatchInput=off
  Reset : Inport  Port=3  LatchInput=off
  Gain1 : Gain  Gain=Time_Const  SaturateOnIntegerOverflow=on
  Random Walk : AeroLib/Sensors/Random Walk  Seed=Seed  Var=Var
  Saturation : Saturate  UpperLimit=Max  LowerLimit=Min
  Stateless_Integrator : AeroLib/AMS_StatelessFilters/Stateless_Integrator
  Sum : Sum  Inputs=|+-  SaturateOnIntegerOverflow=on  InputSameDT=on
  Sum1 : Sum  Inputs=++|  SaturateOnIntegerOverflow=on  InputSameDT=on
  Sen_Out : Outport
  wires:
  Reset/1 -> Stateless_Integrator/1, Random Walk/1
  Random Walk/1 -> Sum1/1
  X0/1 -> Stateless_Integrator/2
  Saturation/1 -> Sum/1
  Stateless_Integrator/1 -> Sum1/2, Sum/2
  Sum/1 -> Gain1/1
  Meas_In/1 -> Saturation/1
  Gain1/1 -> Stateless_Integrator/3
  Sum1/1 -> Sen_Out/1

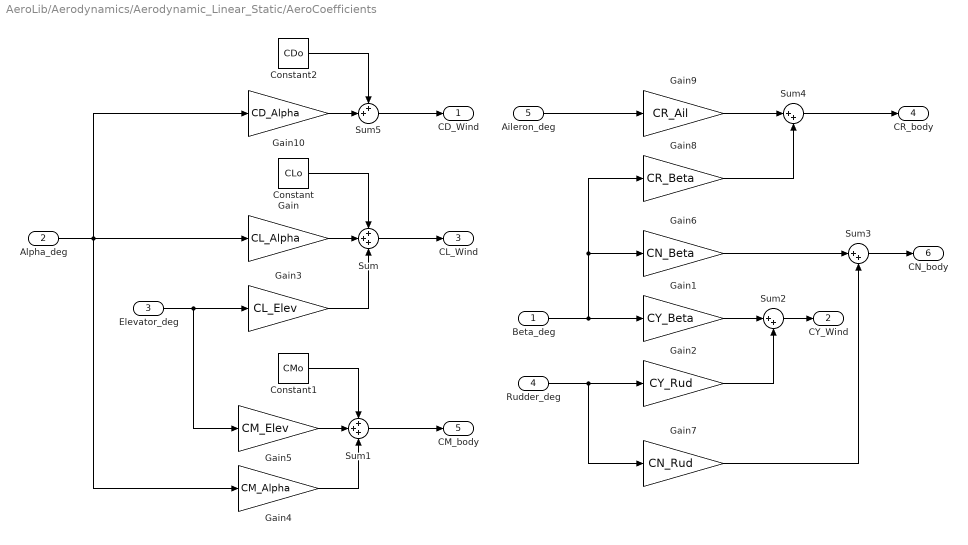
== system AeroLib/Aerodynamics/Aerodynamic_Linear_Static/AeroCoefficients ==
  Beta_deg : Inport  Port=1  LatchInput=off
  Alpha_deg : Inport  Port=2  LatchInput=off
  Elevator_deg : Inport  Port=3  LatchInput=off
  Rudder_deg : Inport  Port=4  LatchInput=off
  Aileron_deg : Inport  Port=5  LatchInput=off
  Constant : Constant  Value=CLo
  Constant1 : Constant  Value=CMo
  Constant2 : Constant  Value=CDo
  Gain : Gain  Gain=CL_Alpha  SaturateOnIntegerOverflow=on
  Gain1 : Gain  Gain=CY_Beta  SaturateOnIntegerOverflow=on
  Gain10 : Gain  Gain=CD_Alpha  SaturateOnIntegerOverflow=on
  Gain2 : Gain  Gain=CY_Rud  SaturateOnIntegerOverflow=on
  Gain3 : Gain  Gain=CL_Elev  SaturateOnIntegerOverflow=on
  Gain4 : Gain  Gain=CM_Alpha  SaturateOnIntegerOverflow=on
  Gain5 : Gain  Gain=CM_Elev  SaturateOnIntegerOverflow=on
  Gain6 : Gain  Gain=CN_Beta  SaturateOnIntegerOverflow=on
  Gain7 : Gain  Gain=CN_Rud  SaturateOnIntegerOverflow=on
  Gain8 : Gain  Gain=CR_Beta  SaturateOnIntegerOverflow=on
  Gain9 : Gain  Gain=CR_Ail  SaturateOnIntegerOverflow=on
  Sum : Sum  Inputs=+++  SaturateOnIntegerOverflow=on
  Sum1 : Sum  Inputs=+++  SaturateOnIntegerOverflow=on
  Sum2 : Sum  Inputs=|++  SaturateOnIntegerOverflow=on
  Sum3 : Sum  Inputs=|++  SaturateOnIntegerOverflow=on
  Sum4 : Sum  Inputs=|++  SaturateOnIntegerOverflow=on
  Sum5 : Sum  Inputs=++|  SaturateOnIntegerOverflow=on
  CD_Wind : Outport
  CY_Wind : Outport  Port=2
  CL_Wind : Outport  Port=3
  CR_body : Outport  Port=4
  CM_body : Outport  Port=5
  CN_body : Outport  Port=6
  wires:
  Constant2/1 -> Sum5/1
  Gain10/1 -> Sum5/2
  Sum5/1 -> CD_Wind/1
  Sum2/1 -> CY_Wind/1
  Sum4/1 -> CR_body/1
  Sum3/1 -> CN_body/1
  Gain9/1 -> Sum4/1
  Gain8/1 -> Sum4/2
  Aileron_deg/1 -> Gain9/1
  Gain7/1 -> Sum3/2
  Gain6/1 -> Sum3/1
  Gain2/1 -> Sum2/2
  Rudder_deg/1 -> Gain7/1, Gain2/1
  Gain1/1 -> Sum2/1
  Beta_deg/1 -> Gain6/1, Gain8/1, Gain1/1
  Constant1/1 -> Sum1/1
  Constant/1 -> Sum/1
  Gain3/1 -> Sum/3
  Gain/1 -> Sum/2
  Sum1/1 -> CM_body/1
  Gain4/1 -> Sum1/3
  Gain5/1 -> Sum1/2
  Elevator_deg/1 -> Gain5/1, Gain3/1
  Sum/1 -> CL_Wind/1
  Alpha_deg/1 -> Gain10/1, Gain/1, Gain4/1

== system AeroLib/Aerodynamics/Aerodynamics_Generic/Aero_Loads ==
  From_Drag : Inport  Port=1  LatchInput=off
  From_SideF : Inport  Port=2  LatchInput=off
  From_Lift : Inport  Port=3  LatchInput=off
  From_Roll : Inport  Port=4  LatchInput=off
  From_Pitch : Inport  Port=5  LatchInput=off
  From_Yaw : Inport  Port=6  LatchInput=off
  From_Atmos : Inport  Port=7  LatchInput=off
  dcg2ac : Inport  Port=8  LatchInput=off
  Bus Selector : BusSelector  DialogController=Simulink.DDGSource_Bus  OutputSignals=DynPres_P,Alpha
  Bus Selector1 : BusSelector  DialogController=Simulink.DDGSource_Bus  OutputSignals=CYs
  Bus Selector2 : BusSelector  DialogController=Simulink.DDGSource_Bus  OutputSignals=CLs
  Demux : Demux  Outputs=6
  Loads : AeroLib/Aerodynamics/Loads  Bref=Geom.Wing.bref  Cref=Geom.Wing.cref  Sw=Geom.Wing.sw
  Mux : Mux  Inputs=10
  Mux1 : Mux  Inputs=6
  STA2BOA : AeroLib/CoordinateSystems/STA2BOA
  Transf to CG : AeroLib/Aerodynamics/Transf to CG  Bref=Geom.Wing.bref  Cref=Geom.Wing.cref
  Xaero : Outport
  wires:
  dcg2ac/1 -> Transf to CG/7
  Demux/6 -> Transf to CG/6
  Demux/5 -> Transf to CG/5
  Demux/4 -> Transf to CG/4
  Demux/3 -> Transf to CG/3
  Demux/2 -> Transf to CG/2
  Demux/1 -> Transf to CG/1
  Transf to CG/6 -> Mux/9, Loads/7  "CNcg"
  Transf to CG/5 -> Mux/8, Loads/6  "CMcg"
  Transf to CG/4 -> Mux/7, Loads/5  "CRcg"
  Transf to CG/3 -> Loads/4
  Transf to CG/2 -> Loads/3
  Transf to CG/1 -> Loads/2
  Bus Selector2/1 -> Mux1/3  "<CLs>"
  Bus Selector1/1 -> Mux1/2  "<CYs>"
  From_Drag/1 -> Mux1/1  "CDs"
  Bus Selector/2 -> STA2BOA/2  "<Alpha>"
  From_Atmos/1 -> Bus Selector/1
  STA2BOA/1 -> Demux/1
  Mux1/1 -> STA2BOA/1, Mux/10  "Caero"
  From_Yaw/1 -> Mux1/6  "CNs"
  From_Pitch/1 -> Mux1/5  "CMs"
  From_Roll/1 -> Mux1/4  "CRs"
  From_Lift/1 -> Bus Selector2/1  "CLs"
  From_SideF/1 -> Bus Selector1/1
  Bus Selector/1 -> Loads/1  "<DynPres_P>"
  Loads/1 -> Mux/1  "Xaero"
  Loads/2 -> Mux/2  "Yaero"
  Loads/3 -> Mux/3  "Zaero"
  Loads/4 -> Mux/4  "Laero"
  Loads/5 -> Mux/5  "Maero"
  Loads/6 -> Mux/6  "Naero"
  Mux/1 -> Xaero/1

== system AeroLib/Aerodynamics/Aerodynamics_Generic/Drag ==
  From_Atmos : Inport  Port=1  LatchInput=off
  From_Ctrl : Inport  Port=2  LatchInput=off
  From_Inputs : Inport  Port=3  LatchInput=off
  " (14)" : Product  Inputs=**  SaturateOnIntegerOverflow=on  InputSameDT=on
  " (15)" : Sum  SaturateOnIntegerOverflow=on  InputSameDT=on
  " (15)1" : Sum  SaturateOnIntegerOverflow=on  InputSameDT=on
  " (22)" : Abs  SaturateOnIntegerOverflow=on
  Bus Selector1 : BusSelector  DialogController=Simulink.DDGSource_Bus  OutputSignals=Alpha,Mach,Beta
  Bus Selector2 : BusSelector  DialogController=Simulink.DDGSource_Bus  OutputSignals=Flap_deg
  Bus Selector3 : BusSelector  DialogController=Simulink.DDGSource_Bus  OutputSignals=GearDown
  CD_wbnp : simulink3/Functions & Tables/Interpolation (n-D) using PreLook-Up  numDimsPopupSelect=3  explicitNumDims=2  table=Aero.Drag.CDs  interpMethod=Linear  extrapMethod=Linear  rangeErrorMode=None
  CdLgAlph : simulink3/Functions & Tables/Look-Up Table (2-D)  x="[-15.0 -10.0  -5.0   0.0   5.0  10.0  15.0  20.0]"  y=[0 10 20 35]  t=Aero.Drag.CDlg
  CdLgBeta : Lookup  DialogController=Simulink.DDGSource  InputValues=[0 5 10 15 20 25 30]  OutputValues="[0.0  0.0008  0.0050  0.0110  0.0190  0.0280 0.0300]"  SaturateOnIntegerOverflow=on
  Gain : Gain  Gain=PEG_CDwbnp  SaturateOnIntegerOverflow=on
  PreLook-Up Index Search3 : simulink3/Functions & Tables/PreLook-Up Index Search  bpData=Aero.Drag.Flap  searchMode=Binary Search  cacheBpFlag=off  outputFlag=off  extrapMode=Linear Extrapolation  rangeErrorMode=None
  PreLook-Up Index Search4 : simulink3/Functions & Tables/PreLook-Up Index Search  bpData=Aero.Drag.Mach  searchMode=Binary Search  cacheBpFlag=off  outputFlag=off  extrapMode=Linear Extrapolation  rangeErrorMode=None
  PreLook-Up Index Search5 : simulink3/Functions & Tables/PreLook-Up Index Search  bpData=Aero.Drag.Alpha  searchMode=Binary Search  cacheBpFlag=off  outputFlag=off  extrapMode=Linear Extrapolation  rangeErrorMode=None
  Drag_Out : Outport
  wires:
  Bus Selector3/1 -> " (14)"/2  "<GearDown>"
  " (15)1"/1 -> Drag_Out/1  "CDs"
  CdLgBeta/1 -> " (15)"/2  "CdLgBeta"
  Bus Selector1/3 -> " (22)"/1  "<Beta>"
  " (22)"/1 -> CdLgBeta/1
  From_Inputs/1 -> Bus Selector3/1
  CdLgAlph/1 -> " (15)"/1  "CDlgAlpha"
  " (15)"/1 -> " (14)"/1
  " (14)"/1 -> " (15)1"/2  "CDlg_A"
  PreLook-Up Index Search5/1 -> CD_wbnp/1
  Bus Selector1/2 -> PreLook-Up Index Search4/1  "<Mach>"
  Bus Selector1/1 -> CdLgAlph/1, PreLook-Up Index Search5/1  "<Alpha>"
  Bus Selector2/1 -> CdLgAlph/2, PreLook-Up Index Search3/1  "<Flap_deg>"
  From_Ctrl/1 -> Bus Selector2/1
  From_Atmos/1 -> Bus Selector1/1
  PreLook-Up Index Search4/1 -> CD_wbnp/3
  PreLook-Up Index Search3/1 -> CD_wbnp/2
  CD_wbnp/1 -> Gain/1  "CDs"
  Gain/1 -> " (15)1"/1

== system AeroLib/Aerodynamics/Aerodynamics_Generic/LIft ==
  From_EQM : Inport  Port=1  LatchInput=off
  From_Atmos : Inport  Port=2  LatchInput=off
  From_Ctrl : Inport  Port=3  LatchInput=off
  Bus Selector : BusSelector  DialogController=Simulink.DDGSource_Bus  OutputSignals=Flap_deg
  Bus Selector1 : BusSelector  DialogController=Simulink.DDGSource_Bus  OutputSignals=Alpha,Mach
  CL Tail : Subsystem
  CL_wnbn : simulink3/Functions & Tables/Interpolation (n-D) using PreLook-Up  numDimsPopupSelect=3  explicitNumDims=2  table=Aero.Lift.CLs  interpMethod=Linear  extrapMethod=Linear  rangeErrorMode=None
  Fcn1 : Fcn  Expr=0.6 + 0.14*u(1) + (0.35 - 0.0045*u(1))*u(2)
  Gain1 : Gain  Gain=PEG_CLwbnp  SaturateOnIntegerOverflow=on
  Mux : Mux  Inputs=2
  Mux1 : Mux  Inputs=2
  PreLook-Up Index Search : simulink3/Functions & Tables/PreLook-Up Index Search  bpData=Aero.Lift.Flap  searchMode=Binary Search  cacheBpFlag=off  outputFlag=off  extrapMode=Linear Extrapolation  rangeErrorMode=None
  PreLook-Up Index Search1 : simulink3/Functions & Tables/PreLook-Up Index Search  bpData=Aero.Lift.Mach  searchMode=Binary Search  cacheBpFlag=off  outputFlag=off  extrapMode=Linear Extrapolation  rangeErrorMode=None
  PreLook-Up Index Search2 : simulink3/Functions & Tables/PreLook-Up Index Search  bpData=Aero.Lift.Alpha  searchMode=Binary Search  cacheBpFlag=off  outputFlag=off  extrapMode=Linear Extrapolation  rangeErrorMode=None
  Sum : Sum  Inputs=+|+  SaturateOnIntegerOverflow=on  InputSameDT=on
  Lift_Out : Outport
  wires:
  From_EQM/1 -> CL Tail/4(From_EQM)
  PreLook-Up Index Search/1 -> CL_wnbn/2
  PreLook-Up Index Search2/1 -> CL_wnbn/1
  Sum/1 -> Mux1/2  "CLs"
  Mux1/1 -> Lift_Out/1  "Lift_s"
  CL Tail/1(CL_Tail) -> Mux1/1, Sum/1  "CLt"
  CL_wnbn/1 -> Gain1/1  "CLwn"
  Fcn1/1 -> CL Tail/2(Epsilon)  "Epsilon"
  Mux/1 -> Fcn1/1
  Bus Selector/1 -> Mux/1, PreLook-Up Index Search/1  "<Flap_deg>"
  Bus Selector1/2 -> PreLook-Up Index Search1/1  "<Mach>"
  Bus Selector1/1 -> Mux/2, PreLook-Up Index Search2/1  "<Alpha>"
  From_Atmos/1 -> CL Tail/3(From_Atmos), Bus Selector1/1
  From_Ctrl/1 -> CL Tail/1(From_Inputs), Bus Selector/1
  PreLook-Up Index Search1/1 -> CL_wnbn/3
  Gain1/1 -> Sum/2  "CLwn"

== system AeroLib/Aerodynamics/Aerodynamics_Generic/Pitching Moment ==
  From_Lift : Inport  Port=1  LatchInput=off
  From_Atmos : Inport  Port=2  LatchInput=off
  From_Ctrl : Inport  Port=3  LatchInput=off
  From_Inputs : Inport  Port=4  LatchInput=off
  " (7)" : Product  Inputs=**  SaturateOnIntegerOverflow=on  InputSameDT=on
  Alpha-Flap Interp1 : simulink3/Functions & Tables/Interpolation (n-D) using PreLook-Up  numDimsPopupSelect=2  explicitNumDims=2  table=Aero.Pitch.CmLG  interpMethod=Linear  extrapMethod=Linear  rangeErrorMode=None
  AlphaIndex : simulink3/Functions & Tables/PreLook-Up Index Search  bpData=[-15 -10 15 20]  searchMode=Linear Search  cacheBpFlag=on  outputFlag=off  extrapMode=Linear Extrapolation  rangeErrorMode=None
  Bus Selector : BusSelector  DialogController=Simulink.DDGSource_Bus  OutputSignals=CLt
  Bus Selector1 : BusSelector  DialogController=Simulink.DDGSource_Bus  OutputSignals=Alpha,Mach
  Bus Selector2 : BusSelector  DialogController=Simulink.DDGSource_Bus  OutputSignals=Flap_deg
  Bus Selector3 : BusSelector  DialogController=Simulink.DDGSource_Bus  OutputSignals=GearDown
  CM_wnbn : simulink3/Functions & Tables/Interpolation (n-D) using PreLook-Up  numDimsPopupSelect=3  explicitNumDims=2  table=Aero.Pitch.CMs  interpMethod=Linear  extrapMethod=Linear  rangeErrorMode=None
  Fcn1 : Fcn  Expr=-u(1)*Geom.Htail.lt/Geom.Wing.cref
  Flap2Index : simulink3/Functions & Tables/PreLook-Up Index Search  bpData=Aero.Pitch.Flap  searchMode=Linear Search  cacheBpFlag=on  outputFlag=off  extrapMode=Linear Extrapolation  rangeErrorMode=None
  Gain : Gain  Gain=PEG_CMwbnp  SaturateOnIntegerOverflow=on
  Gain1 : Gain  Gain=PEG_CMht  SaturateOnIntegerOverflow=on
  PreLook-Up Index Search : simulink3/Functions & Tables/PreLook-Up Index Search  bpData=Aero.Pitch.Flap  searchMode=Binary Search  cacheBpFlag=off  outputFlag=off  extrapMode=Linear Extrapolation  rangeErrorMode=None
  PreLook-Up Index Search1 : simulink3/Functions & Tables/PreLook-Up Index Search  bpData=Aero.Pitch.Mach  searchMode=Binary Search  cacheBpFlag=off  outputFlag=off  extrapMode=Linear Extrapolation  rangeErrorMode=None
  PreLook-Up Index Search2 : simulink3/Functions & Tables/PreLook-Up Index Search  bpData=Aero.Pitch.Alpha  searchMode=Binary Search  cacheBpFlag=off  outputFlag=off  extrapMode=Linear Extrapolation  rangeErrorMode=None
  Sum : Sum  Inputs=+|+|+  SaturateOnIntegerOverflow=on  InputSameDT=on
  PitchM_Out : Outport
  wires:
  Bus Selector3/1 -> " (7)"/2  "<GearDown>"
  " (7)"/1 -> Sum/3
  From_Inputs/1 -> Bus Selector3/1
  Alpha-Flap Interp1/1 -> " (7)"/1
  AlphaIndex/1 -> Alpha-Flap Interp1/1
  Flap2Index/1 -> Alpha-Flap Interp1/2
  Sum/1 -> PitchM_Out/1  "CMs"
  CM_wnbn/1 -> Gain/1  "CMwbn"
  Fcn1/1 -> Gain1/1  "CMt"
  Bus Selector1/2 -> PreLook-Up Index Search1/1  "<Mach>"
  Bus Selector1/1 -> AlphaIndex/1, PreLook-Up Index Search2/1  "<Alpha>"
  Bus Selector/1 -> Fcn1/1  "<CLt>"
  Bus Selector2/1 -> Flap2Index/1, PreLook-Up Index Search/1  "<Flap_deg>"
  From_Ctrl/1 -> Bus Selector2/1
  From_Atmos/1 -> Bus Selector1/1
  From_Lift/1 -> Bus Selector/1
  PreLook-Up Index Search2/1 -> CM_wnbn/1
  PreLook-Up Index Search1/1 -> CM_wnbn/3
  PreLook-Up Index Search/1 -> CM_wnbn/2
  Gain/1 -> Sum/1  "CMwbn"
  Gain1/1 -> Sum/2  "CMt"

== system AeroLib/Aerodynamics/Aerodynamics_Generic/Rolling Moment ==
  From_Ctrl : Inport  Port=1  LatchInput=off
  From_Atmos : Inport  Port=2  LatchInput=off
  From_SideF : Inport  Port=3  LatchInput=off
  Bus Selector : BusSelector  DialogController=Simulink.DDGSource_Bus  OutputSignals=Beta
  Bus Selector1 : BusSelector  DialogController=Simulink.DDGSource_Bus  OutputSignals=Ail_deg,Rud_deg
  Bus Selector2 : BusSelector  DialogController=Simulink.DDGSource_Bus  OutputSignals=phat
  Fcn1 : Fcn  Expr=0.002*u(1)
  Fcn2 : Fcn  Expr=0.0012*u(1)
  Fcn3 : Fcn  Expr=-.55*u(1)
  Fcn4 : Fcn  Expr=-.0012*u(1)
  Gain : Gain  Gain=PEG_CRrud  SaturateOnIntegerOverflow=on
  Gain1 : Gain  Gain=PEG_CRbeta  SaturateOnIntegerOverflow=on
  Gain2 : Gain  Gain=PEG_CRp  SaturateOnIntegerOverflow=on
  Gain3 : Gain  Gain=PEG_CRail  SaturateOnIntegerOverflow=on
  Sum : Sum  Inputs=++++  SaturateOnIntegerOverflow=on  InputSameDT=on
  RollM_Out : Outport
  wires:
  Fcn2/1 -> Gain/1  "CR_Rud"
  Sum/1 -> RollM_Out/1  "CRs"
  Fcn4/1 -> Gain1/1  "CR_Beta"
  Fcn1/1 -> Gain3/1  "CR_Ail"
  Fcn3/1 -> Gain2/1  "CR_P"
  Bus Selector2/1 -> Fcn3/1  "<phat>"
  From_SideF/1 -> Bus Selector2/1
  Bus Selector1/2 -> Fcn2/1  "<Rud_deg>"
  Bus Selector1/1 -> Fcn1/1  "<Ail_deg>"
  Bus Selector/1 -> Fcn4/1  "<Beta>"
  From_Ctrl/1 -> Bus Selector1/1
  From_Atmos/1 -> Bus Selector/1
  Gain/1 -> Sum/3  "CR_Rud"
  Gain1/1 -> Sum/4  "CR_Beta"
  Gain2/1 -> Sum/1  "CR_P"
  Gain3/1 -> Sum/2  "CR_Ail"

== system AeroLib/Aerodynamics/Aerodynamics_Generic/Side Force ==
  From_Ctrl : Inport  Port=1  LatchInput=off
  From_Atmos : Inport  Port=2  LatchInput=off
  From_EQM : Inport  Port=3  LatchInput=off
  Bus Selector : BusSelector  DialogController=Simulink.DDGSource_Bus  OutputSignals=Rud_deg
  Bus Selector1 : BusSelector  DialogController=Simulink.DDGSource_Bus  OutputSignals=Beta,TAS
  Bus Selector2 : BusSelector  DialogController=Simulink.DDGSource_Bus  OutputSignals=P_rad,R_rad
  Fcn1 : Fcn  Expr=u(2)*Geom.Wing.span/(2.0*u(1))
  Fcn2 : Fcn  Expr=u(3)*Geom.Wing.span/(2.0*u(1))
  Fcn3 : Fcn  Expr=0.0024*u(1)
  Fcn4 : Fcn  Expr=-0.013*u(1)
  Fcn5 : Fcn  Expr=0.7*u(1)
  Gain : Gain  Gain=PEG_CYrud  SaturateOnIntegerOverflow=on
  Gain1 : Gain  Gain=PEG_CYbeta  SaturateOnIntegerOverflow=on
  Mux : Mux  Inputs=3
  Mux1 : Mux  Inputs=3
  Sum : Sum  Inputs=+++  SaturateOnIntegerOverflow=on  InputSameDT=on
  SideF_Out : Outport
  wires:
  Mux1/1 -> SideF_Out/1  "SideF"
  Sum/1 -> Mux1/1  "CYs"
  Fcn5/1 -> Sum/3  "CY_R"
  Fcn4/1 -> Gain1/1  "CY_Beta"
  Fcn3/1 -> Gain/1  "CY_Rud"
  Fcn2/1 -> Mux1/3, Fcn5/1  "rhat"
  Fcn1/1 -> Mux1/2  "phat"
  Mux/1 -> Fcn2/1, Fcn1/1
  Bus Selector2/2 -> Mux/3  "<R_rad>"
  Bus Selector2/1 -> Mux/2  "<P_rad>"
  Bus Selector1/2 -> Mux/1  "<TAS>"
  Bus Selector1/1 -> Fcn4/1  "<Beta>"
  Bus Selector/1 -> Fcn3/1  "<Rud_deg>"
  From_EQM/1 -> Bus Selector2/1
  From_Atmos/1 -> Bus Selector1/1
  From_Ctrl/1 -> Bus Selector/1
  Gain/1 -> Sum/1  "CY_Rud"
  Gain1/1 -> Sum/2  "CY_Beta"

== system AeroLib/Aerodynamics/Aerodynamics_Generic/Yawing Moment ==
  From_SideF : Inport  Port=1  LatchInput=off
  From_Ctrl : Inport  Port=2  LatchInput=off
  From_Atmos : Inport  Port=3  LatchInput=off
  Bus Selector1 : BusSelector  DialogController=Simulink.DDGSource_Bus  OutputSignals=rhat
  Bus Selector2 : BusSelector  DialogController=Simulink.DDGSource_Bus  OutputSignals=Rud_deg
  Bus Selector3 : BusSelector  DialogController=Simulink.DDGSource_Bus  OutputSignals=Beta
  Fcn1 : Fcn  Expr=-0.4*u(1)
  Fcn2 : Fcn  Expr=0.0022*u(1)
  Fcn4 : Fcn  Expr=-0.0027*u(1)
  Gain : Gain  Gain=PEG_CNrud  SaturateOnIntegerOverflow=on
  Gain1 : Gain  Gain=PEG_CNr  SaturateOnIntegerOverflow=on
  Gain2 : Gain  Gain=PEG_CNbeta  SaturateOnIntegerOverflow=on
  Sum : Sum  Inputs=+++  SaturateOnIntegerOverflow=on  InputSameDT=on
  YawM_Out : Outport
  wires:
  Sum/1 -> YawM_Out/1  "CNs"
  Fcn2/1 -> Gain2/1  "CN_Beta"
  Fcn1/1 -> Gain1/1  "CN_R"
  Bus Selector1/1 -> Fcn1/1  "<rhat>"
  Fcn4/1 -> Gain/1  "CN_Rud"
  Bus Selector3/1 -> Fcn2/1  "<Beta>"
  Bus Selector2/1 -> Fcn4/1  "<Rud_deg>"
  From_Ctrl/1 -> Bus Selector2/1
  From_SideF/1 -> Bus Selector1/1
  From_Atmos/1 -> Bus Selector3/1
  Gain/1 -> Sum/1  "CN_Rud"
  Gain1/1 -> Sum/2  "CN_R"
  Gain2/1 -> Sum/3  "CN_Beta"
